simulink model "NL_Corner"  (R2016b)
settings: Solver=FixedStepAuto  StartTime=0.0  StopTime=100  FixedStep=0.001  RelTol=1e-3
values from neighbouring files (symbols this model uses):
  AccelError = double(subs(A_P_K, phi, degtorad(accelTilt)))    [SimulinkInit.m]
  C_psi = 3.1176e-5    (= 3.1176e-05)    [ParameterInit.m]
  control_system = CS_CompLQR    (= 2)    [SimulinkInit.m]
  dPhiMat = [cos(phi_30)/cos(phi_20), -sin(phi_30)/cos(phi_20), 0 ... (first row only)    [ParameterInit.m]
  g = 9.81    [ParameterInit.m]
  GyroError = double(subs(A_P_K, phi, degtorad(gyroTilt)))    [SimulinkInit.m]
  I_K_inv = inv(I_K)    [ParameterInit.m]
  I_R_inv = inv(I_R)    [ParameterInit.m]
  Kd = K_unlimited    [LinearSimulationScript.m]    (also in controller_design_lqr.m = KKd * [eye(7), zeros(7,2)]/T_K)
  l_C = 0.066    [ParameterInit.m]
  m = 1.532    [ParameterInit.m]
  phi0 = x0(1:3) + [0; phi_20; phi_30]    [SimulinkInit.m]
  phi_20 = -2*atan(sqrt(2)-sqrt(3))    [ParameterInit.m]
  phi_30 = -pi/4    (= -0.785398163397)    [ParameterInit.m]
  Ta = 0.02    [ParameterInit.m]
  u_K0 = x0(4:6)    [SimulinkInit.m]
  u_R0 = x0(7:9)    [SimulinkInit.m]
  x0 = [0; 0.11; 0.08; 0; 1; -2; 3; -16; 0]    [LinearSimulationScript.m]    (also in SimulinkInit.m = [0; 0.01; 0; 0; 0; 0; 0; 0; 0])
  x_offset = [0; 0.02; 0.0; 0; 0; 0; 0; 0; 0]    [SimulinkInit.m]
libraries: simulink x1
settings Model: Creator=michael  LastModifiedBy=michael

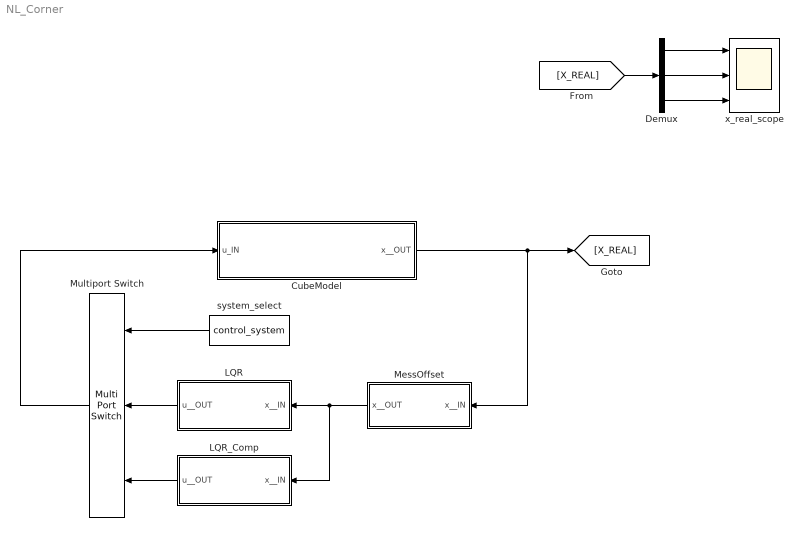
== system NL_Corner ==
  CubeModel : Subsystem
  Demux : Demux  Outputs=3
  LQR : Subsystem
  LQR_Comp : Subsystem
  MessOffset : Subsystem
  Multiport Switch : MultiPortSwitch  Inputs=2
  system_select : Constant  Value=control_system
  x_real_scope : Scope  NumInputPorts=3
  wires:
  MessOffset/1(x__OUT) -> LQR/1(x__IN), LQR_Comp/1(x__IN)
  CubeModel/1(x__OUT) -> [X_REAL], MessOffset/1(x__IN)
  [X_REAL] -> Demux/1
  Demux/1 -> x_real_scope/1
  Demux/2 -> x_real_scope/2
  Demux/3 -> x_real_scope/3
  LQR/1(u__OUT) -> Multiport Switch/2
  LQR_Comp/1(u__OUT) -> Multiport Switch/3
  Multiport Switch/1 -> CubeModel/1(u_IN)
  system_select/1 -> Multiport Switch/1

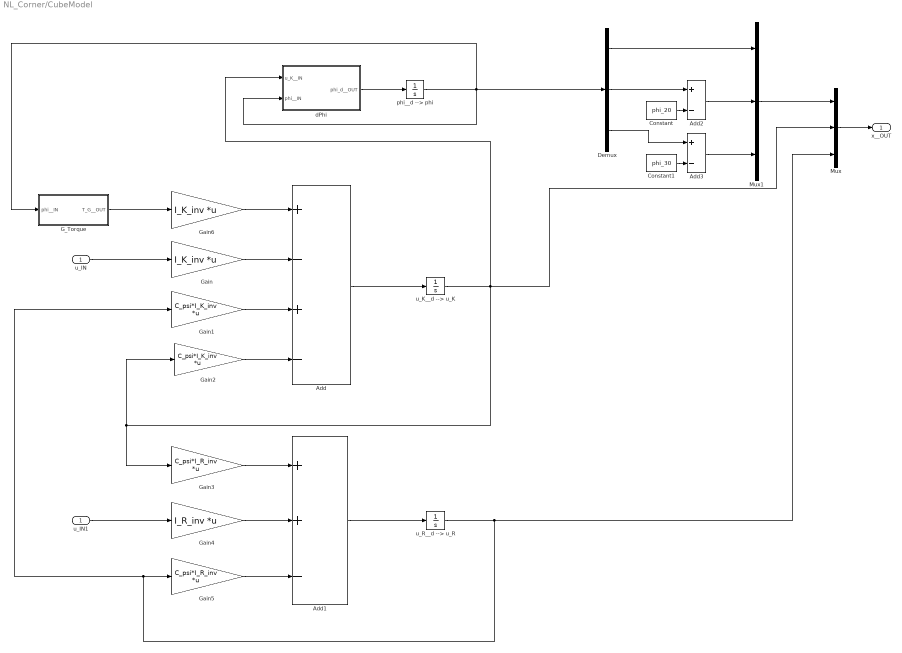
== system NL_Corner/CubeModel ==
  u_IN : Inport
  Add : Sum  Inputs=+-+-
  Add1 : Sum  Inputs=++-
  Add2 : Sum  Inputs=+-
  Add3 : Sum  Inputs=+-
  Constant : Constant  Value=phi_20
  Constant1 : Constant  Value=phi_30
  Demux : Demux  Outputs=3
  G_Torque : Subsystem
  Gain : Gain  Gain=I_K_inv  Multiplication=Matrix(K*u) (u vector)
  Gain1 : Gain  Gain=C_psi*I_K_inv  Multiplication=Matrix(K*u) (u vector)
  Gain2 : Gain  Gain=C_psi*I_K_inv  Multiplication=Matrix(K*u) (u vector)
  Gain3 : Gain  Gain=C_psi*I_R_inv  Multiplication=Matrix(K*u) (u vector)
  Gain4 : Gain  Gain=I_R_inv  Multiplication=Matrix(K*u) (u vector)
  Gain5 : Gain  Gain=C_psi*I_R_inv  Multiplication=Matrix(K*u) (u vector)
  Gain6 : Gain  Gain=I_K_inv  Multiplication=Matrix(K*u)
  Mux : Mux  Inputs=3
  Mux1 : Mux  Inputs=3
  dPhi : Subsystem
  phi__d --> phi : Integrator  InitialCondition=phi0
  u_IN1 : InportShadow
  u_K__d --> u_K : Integrator  InitialCondition=u_K0
  u_R__d --> u_R : Integrator  InitialCondition=u_R0
  x__OUT : Outport
  wires:
  Add/1 -> u_K__d --> u_K/1
  G_Torque/1(T_G__OUT) -> Gain6/1
  Gain/1 -> Add/2
  u_IN/1 -> Gain/1
  Gain1/1 -> Add/3
  Gain2/1 -> Add/4
  u_K__d --> u_K/1 -> Gain3/1, Gain2/1, dPhi/1(u_K__IN), Mux/2
  Gain3/1 -> Add1/1
  Gain4/1 -> Add1/2
  u_IN1/1 -> Gain4/1
  Add1/1 -> u_R__d --> u_R/1
  Gain5/1 -> Add1/3
  u_R__d --> u_R/1 -> Mux/3, Gain5/1, Gain1/1
  dPhi/1(phi_d__OUT) -> phi__d --> phi/1
  Gain6/1 -> Add/1
  Mux/1 -> x__OUT/1
  phi__d --> phi/1 -> G_Torque/1(phi__IN), Demux/1, dPhi/2(phi__IN)
  Demux/2 -> Add2/1
  Demux/3 -> Add3/1
  Constant1/1 -> Add3/2
  Constant/1 -> Add2/2
  Demux/1 -> Mux1/1
  Add2/1 -> Mux1/2
  Add3/1 -> Mux1/3
  Mux1/1 -> Mux/1

== system NL_Corner/LQR ==
  x__IN : Inport  SampleTime=Ta
  Gain : Gain  Gain=-Kd  Multiplication=Matrix(K*u) (u vector)
  u__OUT : Outport
  wires:
  x__IN/1 -> Gain/1
  Gain/1 -> u__OUT/1

== system NL_Corner/LQR_Comp ==
  x__IN : Inport  SampleTime=Ta
  CompFilter : Subsystem
  Gain : Gain  Gain=-Kd  Multiplication=Matrix(K*u) (u vector)
  u__OUT : Outport
  wires:
  x__IN/1 -> CompFilter/1(x__IN)
  Gain/1 -> u__OUT/1
  CompFilter/1(x__OUT) -> Gain/1

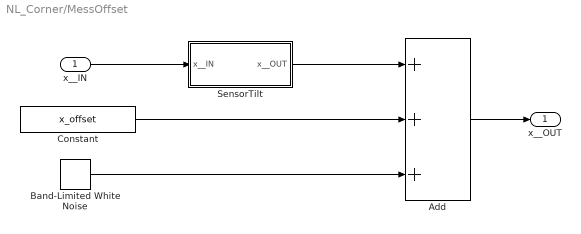
== system NL_Corner/MessOffset ==
  x__IN : Inport
  Add : Sum  Inputs=+++
  Band-Limited White Noise : simulink/Sources/Band-Limited White Noise  Cov=x_noise  Ts=0.1  seed=[1;2;3;4;5;6;7;8;9]
  Constant : Constant  Value=x_offset
  SensorTilt : Subsystem
  x__OUT : Outport
  wires:
  x__IN/1 -> SensorTilt/1(x__IN)
  Add/1 -> x__OUT/1
  Constant/1 -> Add/2
  Band-Limited White Noise/1 -> Add/3
  SensorTilt/1(x__OUT) -> Add/1

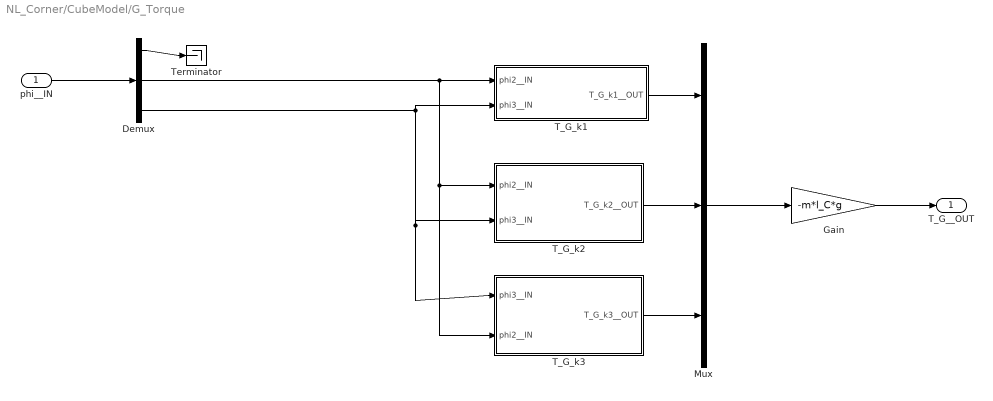
== system NL_Corner/CubeModel/G_Torque ==
  phi__IN : Inport
  Demux : Demux  Outputs=3
  Gain : Gain  Gain=-m*l_C*g
  Mux : Mux  Inputs=3
  T_G_k1 : Subsystem
  T_G_k2 : Subsystem
  T_G_k3 : Subsystem
  Terminator : Terminator
  T_G__OUT : Outport
  wires:
  phi__IN/1 -> Demux/1
  Demux/1 -> Terminator/1
  Demux/2 -> T_G_k3/2(phi2__IN), T_G_k2/1(phi2__IN), T_G_k1/1(phi2__IN)
  Demux/3 -> T_G_k3/1(phi3__IN), T_G_k2/2(phi3__IN), T_G_k1/2(phi3__IN)
  T_G_k3/1(T_G_k3__OUT) -> Mux/3
  Mux/1 -> Gain/1
  T_G_k2/1(T_G_k2__OUT) -> Mux/2
  T_G_k1/1(T_G_k1__OUT) -> Mux/1
  Gain/1 -> T_G__OUT/1

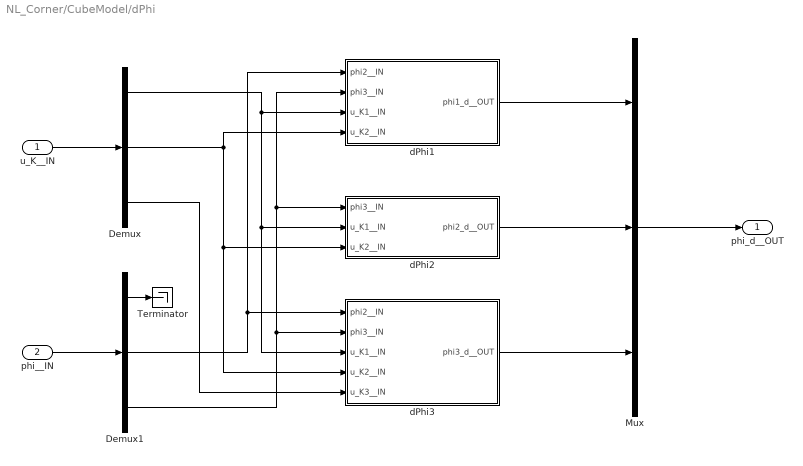
== system NL_Corner/CubeModel/dPhi ==
  u_K__IN : Inport
  phi__IN : Inport  Port=2
  Demux : Demux  Outputs=3
  Demux1 : Demux  Outputs=3
  Mux : Mux  Inputs=3
  Terminator : Terminator
  dPhi1 : Subsystem
  dPhi2 : Subsystem
  dPhi3 : Subsystem
  phi_d__OUT : Outport
  wires:
  u_K__IN/1 -> Demux/1
  Mux/1 -> phi_d__OUT/1
  phi__IN/1 -> Demux1/1
  dPhi1/1(phi1_d__OUT) -> Mux/1
  dPhi2/1(phi2_d__OUT) -> Mux/2
  dPhi3/1(phi3_d__OUT) -> Mux/3
  Demux1/2 -> dPhi3/1(phi2__IN), dPhi1/1(phi2__IN)
  Demux1/3 -> dPhi3/2(phi3__IN), dPhi2/1(phi3__IN), dPhi1/2(phi3__IN)
  Demux1/1 -> Terminator/1
  Demux/2 -> dPhi2/3(u_K2__IN), dPhi3/4(u_K2__IN), dPhi1/4(u_K2__IN)
  Demux/3 -> dPhi3/5(u_K3__IN)
  Demux/1 -> dPhi1/3(u_K1__IN), dPhi2/2(u_K1__IN), dPhi3/3(u_K1__IN)

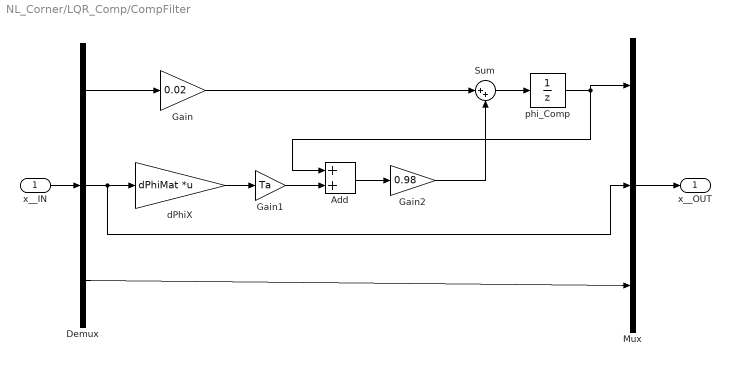
== system NL_Corner/LQR_Comp/CompFilter ==
  x__IN : Inport
  Add : Sum
  Demux : Demux  Outputs=3
  Gain : Gain  Gain=0.02
  Gain1 : Gain  Gain=Ta
  Gain2 : Gain  Gain=0.98
  Mux : Mux  Inputs=3
  Sum : Sum  Inputs=|++
  dPhiX : Gain  Gain=dPhiMat  Multiplication=Matrix(K*u) (u vector)
  phi_Comp : UnitDelay  InitialCondition=x0(1:3)  SampleTime=0.02
  x__OUT : Outport
  wires:
  x__IN/1 -> Demux/1
  Demux/1 -> Gain/1
  Demux/2 -> Mux/2, dPhiX/1
  dPhiX/1 -> Gain1/1
  Gain1/1 -> Add/2
  Add/1 -> Gain2/1
  Gain/1 -> Sum/1
  Gain2/1 -> Sum/2
  Sum/1 -> phi_Comp/1
  phi_Comp/1 -> Add/1, Mux/1
  Mux/1 -> x__OUT/1
  Demux/3 -> Mux/3

== system NL_Corner/MessOffset/SensorTilt ==
  x__IN : Inport
  Demux : Demux  Outputs=3
  Gain : Gain  Gain=GyroError  Multiplication=Matrix(K*u) (u vector)
  Gain1 : Gain  Gain=AccelError  Multiplication=Matrix(K*u) (u vector)
  Mux : Mux  Inputs=3
  x__OUT : Outport
  wires:
  x__IN/1 -> Demux/1
  Demux/2 -> Gain/1
  Mux/1 -> x__OUT/1
  Gain/1 -> Mux/2
  Demux/1 -> Gain1/1
  Demux/3 -> Mux/3
  Gain1/1 -> Mux/1

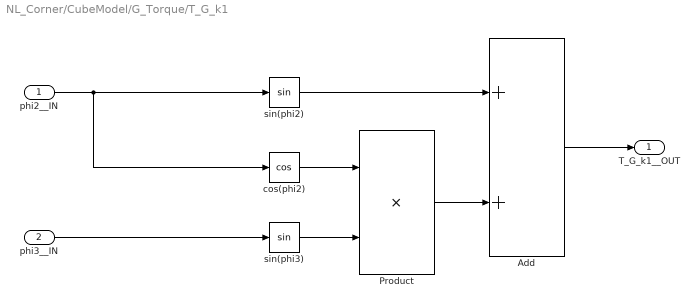
== system NL_Corner/CubeModel/G_Torque/T_G_k1 ==
  phi2__IN : Inport
  phi3__IN : Inport  Port=2
  Add : Sum
  Product : Product
  cos(phi2) : Trigonometry  Operator=cos
  sin(phi2) : Trigonometry
  sin(phi3) : Trigonometry
  T_G_k1__OUT : Outport
  wires:
  phi2__IN/1 -> cos(phi2)/1, sin(phi2)/1
  cos(phi2)/1 -> Product/1
  sin(phi2)/1 -> Add/1
  Product/1 -> Add/2
  phi3__IN/1 -> sin(phi3)/1
  sin(phi3)/1 -> Product/2
  Add/1 -> T_G_k1__OUT/1

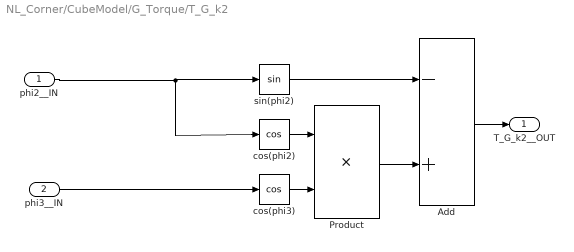
== system NL_Corner/CubeModel/G_Torque/T_G_k2 ==
  phi2__IN : Inport
  phi3__IN : Inport  Port=2
  Add : Sum  Inputs=-+
  Product : Product
  cos(phi2) : Trigonometry  Operator=cos
  cos(phi3) : Trigonometry  Operator=cos
  sin(phi2) : Trigonometry
  T_G_k2__OUT : Outport
  wires:
  sin(phi2)/1 -> Add/1
  phi2__IN/1 -> cos(phi2)/1, sin(phi2)/1
  cos(phi2)/1 -> Product/1
  Add/1 -> T_G_k2__OUT/1
  phi3__IN/1 -> cos(phi3)/1
  cos(phi3)/1 -> Product/2
  Product/1 -> Add/2

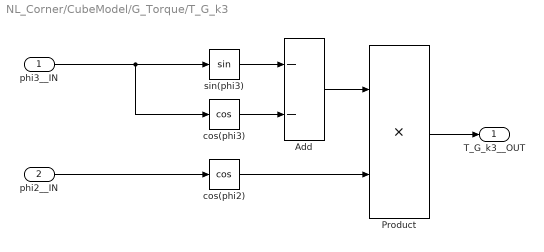
== system NL_Corner/CubeModel/G_Torque/T_G_k3 ==
  phi3__IN : Inport
  phi2__IN : Inport  Port=2
  Add : Sum  Inputs=--
  Product : Product
  cos(phi2) : Trigonometry  Operator=cos
  cos(phi3) : Trigonometry  Operator=cos
  sin(phi3) : Trigonometry
  T_G_k3__OUT : Outport
  wires:
  Product/1 -> T_G_k3__OUT/1
  phi3__IN/1 -> cos(phi3)/1, sin(phi3)/1
  phi2__IN/1 -> cos(phi2)/1
  cos(phi3)/1 -> Add/2
  cos(phi2)/1 -> Product/2
  sin(phi3)/1 -> Add/1
  Add/1 -> Product/1

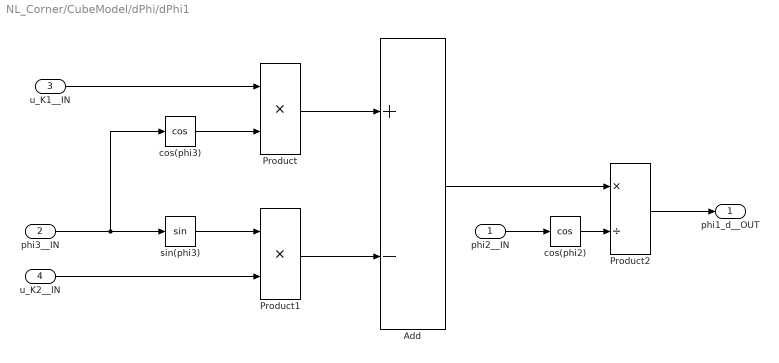
== system NL_Corner/CubeModel/dPhi/dPhi1 ==
  phi2__IN : Inport
  phi3__IN : Inport  Port=2
  u_K1__IN : Inport  Port=3
  u_K2__IN : Inport  Port=4
  Add : Sum  Inputs=+-
  Product : Product  Inputs=**
  Product1 : Product  Inputs=**
  Product2 : Product  Inputs=*/
  cos(phi2) : Trigonometry  Operator=cos
  cos(phi3) : Trigonometry  Operator=cos
  sin(phi3) : Trigonometry
  phi1_d__OUT : Outport
  wires:
  phi3__IN/1 -> cos(phi3)/1, sin(phi3)/1
  cos(phi3)/1 -> Product/2
  u_K1__IN/1 -> Product/1
  sin(phi3)/1 -> Product1/1
  u_K2__IN/1 -> Product1/2
  Product/1 -> Add/1
  Product1/1 -> Add/2
  phi2__IN/1 -> cos(phi2)/1
  Add/1 -> Product2/1
  cos(phi2)/1 -> Product2/2
  Product2/1 -> phi1_d__OUT/1

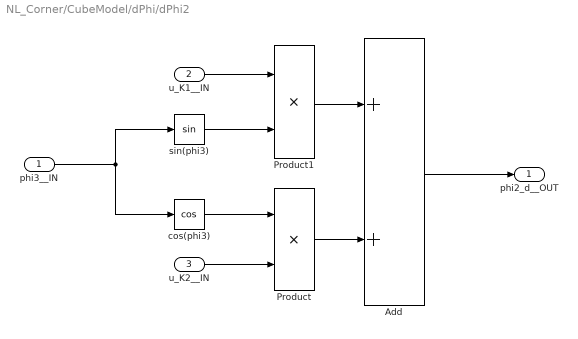
== system NL_Corner/CubeModel/dPhi/dPhi2 ==
  phi3__IN : Inport
  u_K1__IN : Inport  Port=2
  u_K2__IN : Inport  Port=3
  Add : Sum
  Product : Product
  Product1 : Product
  cos(phi3) : Trigonometry  Operator=cos
  sin(phi3) : Trigonometry
  phi2_d__OUT : Outport
  wires:
  phi3__IN/1 -> sin(phi3)/1, cos(phi3)/1
  cos(phi3)/1 -> Product/1
  u_K2__IN/1 -> Product/2
  u_K1__IN/1 -> Product1/1
  sin(phi3)/1 -> Product1/2
  Product1/1 -> Add/1
  Product/1 -> Add/2
  Add/1 -> phi2_d__OUT/1

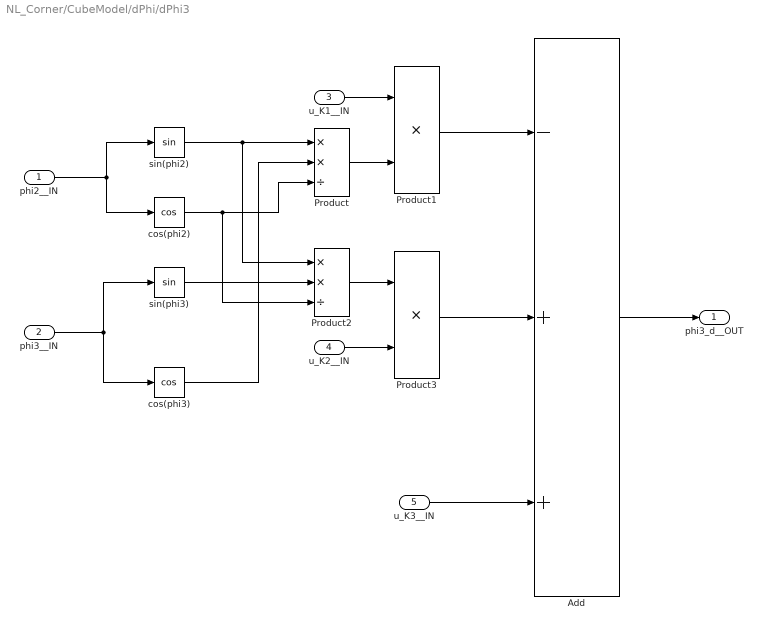
== system NL_Corner/CubeModel/dPhi/dPhi3 ==
  phi2__IN : Inport
  phi3__IN : Inport  Port=2
  u_K1__IN : Inport  Port=3
  u_K2__IN : Inport  Port=4
  u_K3__IN : Inport  Port=5
  Add : Sum  Inputs=-++
  Product : Product  Inputs=**/
  Product1 : Product
  Product2 : Product  Inputs=**/
  Product3 : Product
  cos(phi2) : Trigonometry  Operator=cos
  cos(phi3) : Trigonometry  Operator=cos
  sin(phi2) : Trigonometry
  sin(phi3) : Trigonometry
  phi3_d__OUT : Outport
  wires:
  phi2__IN/1 -> cos(phi2)/1, sin(phi2)/1
  phi3__IN/1 -> cos(phi3)/1, sin(phi3)/1
  sin(phi2)/1 -> Product2/1, Product/1
  cos(phi3)/1 -> Product/2
  u_K1__IN/1 -> Product1/1
  Product/1 -> Product1/2
  cos(phi2)/1 -> Product2/3, Product/3
  sin(phi3)/1 -> Product2/2
  Product2/1 -> Product3/1
  u_K2__IN/1 -> Product3/2
  Product1/1 -> Add/1
  Product3/1 -> Add/2
  u_K3__IN/1 -> Add/3
  Add/1 -> phi3_d__OUT/1
